simulink model "run_bota_ethercat_2020a"  (R2020a)
settings: Solver=ode5  StartTime=0.0  StopTime=inf  FixedStep=0.001  RelTol=1e-3
settings Model: Creator=Martin Wermelinger  LastModifiedBy=Martin Wermelinger
settings DebuggingCC: SFMachineParentedDataDiag=error
settings RTWCC: Description=Generic Real-Time Target
settings CodeAppCC: MaxIdLength=95

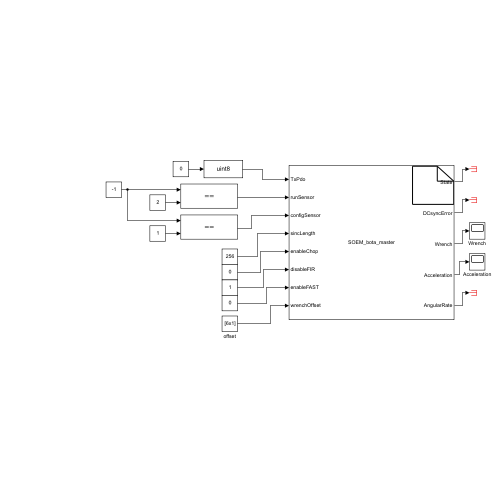
[thumbnail: Simulink's stored preview of the top-level diagram]
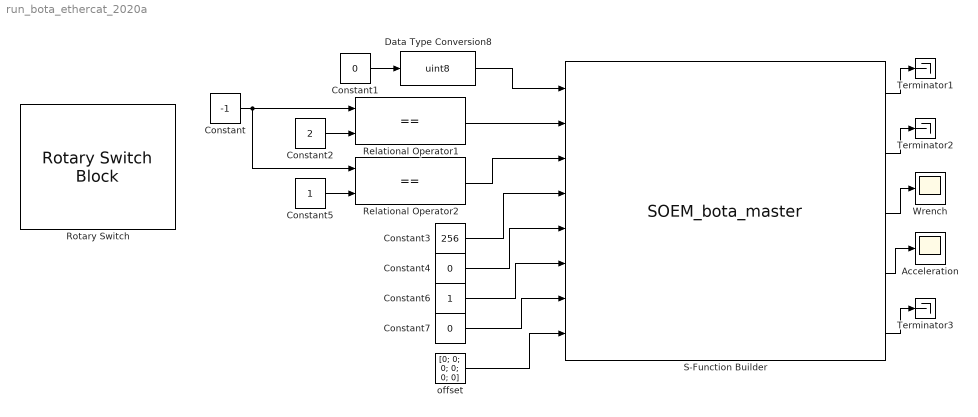
== system run_bota_ethercat_2020a ==
  Acceleration : Scope
  Constant : Constant  Value=-1  SampleTime=-1
  Constant1 : Constant  Value=0  SampleTime=0.001
  Constant2 : Constant  Value=2  SampleTime=-1
  Constant3 : Constant  Value=256  OutDataTypeStr=uint16  SampleTime=-1
  Constant4 : Constant  Value=0  OutDataTypeStr=uint8  SampleTime=-1
  Constant5 : Constant  SampleTime=-1
  Constant6 : Constant  OutDataTypeStr=uint8  SampleTime=-1
  Constant7 : Constant  Value=0  OutDataTypeStr=uint8  SampleTime=-1
  Data Type Conversion8 : DataTypeConversion  OutDataTypeStr=uint8
  Relational Operator1 : RelationalOperator  Operator===  OutDataTypeStr=boolean  RndMeth=Simplest
  Relational Operator2 : RelationalOperator  Operator===  OutDataTypeStr=boolean  RndMeth=Simplest
  Rotary Switch : RotarySwitchBlock
      settings: Values={{'Stop', 'Config', 'Run'}, [-1 1 2]}
  S-Function Builder : S-Function  FunctionName=SOEM_bota_master  Parameters=7,0,0  SFunctionModules=SOEM_bota_master_wrapper  SFunctionDeploymentMode=off  EnableBusSupport=off  mask(S-Function Builder){}
      mask help: Simulink:masks:SFunctionBuilder_MD
      mask init:
      | val = [[.9  0.75 0.75 1 1 .9 .9 1]',[1 1 0.75 0.75 .9 .9 1 .9]'];try , sys = get_param(gcb,'SfunBuilderFcnName');if isempty(sys), sys = get_param(gcb,'FunctionName'); end,catch, sys = get_param(gcb,'FunctionName'); end
      settings: CopyFcn=set_param(gcbh,'LinkStatus','none')  OpenFcn=sfunctionwizard(gcbh)
      mask Display: plot(val(:,1),val(:,2)),disp(sys),port_label('input',1,'TxPdo'),port_label('input',2,'runSensor'),port_label('input',3,'configSensor'),port_label('input',4,'sincLength'),port_label('input',5,'enableChop'),port_label('input',6,'disableFIR'),port_label('input',7,'enableFAST'),port_label('input',8,'wrenchOffset'),port_label('output',1,'State'),port_label('output',2,'DCsyncError'),port_label('output',3,'Wrench'),port_label('output',4,'Acceleration'),port_label('output',5,'AngularRate')
  Terminator1 : Terminator
  Terminator2 : Terminator
  Terminator3 : Terminator
  Wrench : Scope
  offset : Constant  Value=[0; 0; 0; 0; 0; 0]  OutDataTypeStr=single  SampleTime=-1
  wires:
  Constant2/1 -> Relational Operator1/2
  Relational Operator1/1 -> S-Function Builder/2
  Constant1/1 -> Data Type Conversion8/1
  Data Type Conversion8/1 -> S-Function Builder/1
  S-Function Builder/1 -> Terminator1/1
  S-Function Builder/2 -> Terminator2/1
  S-Function Builder/5 -> Terminator3/1
  S-Function Builder/3 -> Wrench/1
  S-Function Builder/4 -> Acceleration/1
  Constant5/1 -> Relational Operator2/2
  Constant/1 -> Relational Operator2/1, Relational Operator1/1
  Relational Operator2/1 -> S-Function Builder/3
  Constant6/1 -> S-Function Builder/6
  Constant3/1 -> S-Function Builder/4
  Constant7/1 -> S-Function Builder/7
  Constant4/1 -> S-Function Builder/5
  offset/1 -> S-Function Builder/8
